simulink model "B3_2D_quadcopter_model"  (R2021b)
settings: Solver=VariableStepAuto  StartTime=0.0  StopTime=10  RelTol=1e-3
values from neighbouring files (symbols this model uses):
  omega_c_motors = 50    [A11_setup_script_pprz.m]    (also in A1_setup_script.m)
libraries: dspinverses x2, sim3dlib x1, uavsim3dlib x1, vrlib x1
settings Model: Creator=pieca  LastModifiedBy=pieca

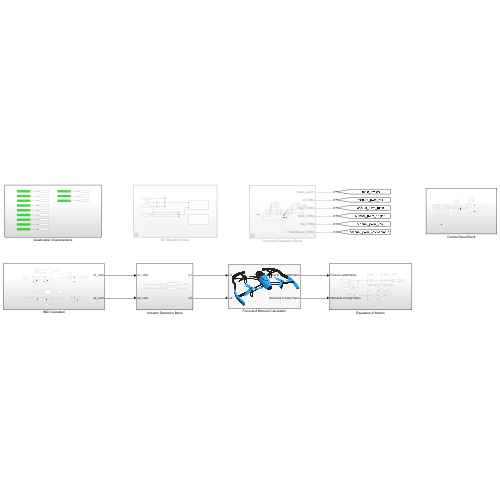
[thumbnail: Simulink's stored preview of the top-level diagram]
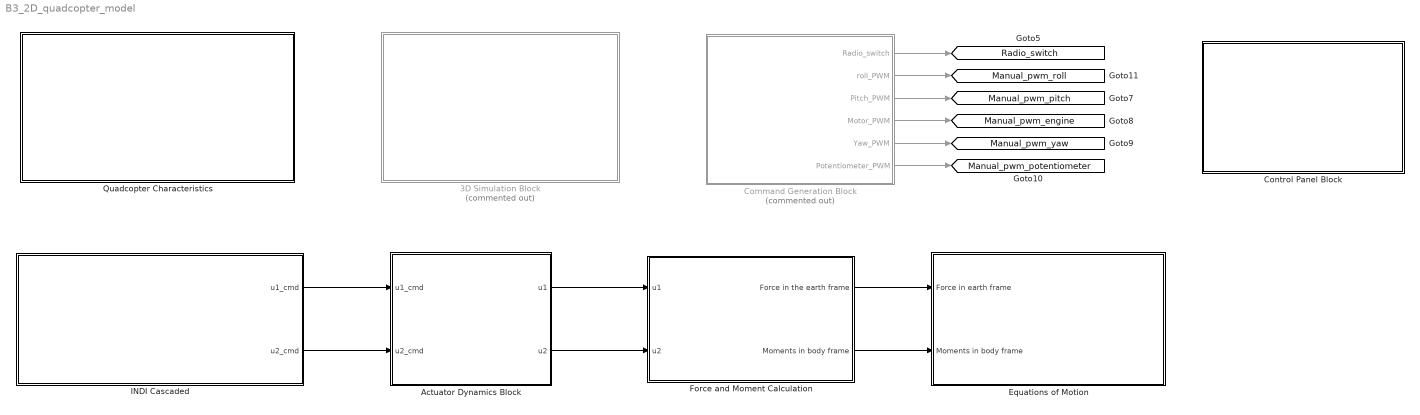
== system B3_2D_quadcopter_model ==
  3D Simulation Block : Subsystem  Commented=on
  Actuator Dynamics Block : Subsystem
  Command Generation Block : Subsystem  Commented=on
  Control Panel Block : Subsystem
  Equations of Motion : Subsystem
  Force and Moment Calculation : Subsystem
      mask Display: image('C:\Users\pieca\Desktop\AE5310-Thesis-Control\Quadcopter\media\bebop.jpg'); % Use "Edit Image" on toolstrip to change.
  INDI Cascaded : Subsystem
  Quadcopter Characteristics : Subsystem
  tag scope: Manual_pwm_engine=global, Manual_pwm_pitch=global, Manual_pwm_potentiometer=global, Manual_pwm_roll=global, Manual_pwm_yaw=global, Radio_switch=global
  wires:
  Command Generation Block/1(Radio_switch) -> [Radio_switch]
  Command Generation Block/2(roll_PWM) -> [Manual_pwm_roll]
  Command Generation Block/3(Pitch_PWM) -> [Manual_pwm_pitch]
  Command Generation Block/4(Motor_PWM) -> [Manual_pwm_engine]
  Command Generation Block/5(Yaw_PWM) -> [Manual_pwm_yaw]
  Command Generation Block/6(Potentiometer_PWM) -> [Manual_pwm_potentiometer]
  Force and Moment Calculation/1(Force in the earth frame) -> Equations of Motion/1(Force in earth frame)
  Force and Moment Calculation/2(Moments in body frame) -> Equations of Motion/2(Moments in body frame)
  Actuator Dynamics Block/1(u1) -> Force and Moment Calculation/1(u1)
  Actuator Dynamics Block/2(u2) -> Force and Moment Calculation/2(u2)
  INDI Cascaded/1(u1_cmd) -> Actuator Dynamics Block/1(u1_cmd)
  INDI Cascaded/2(u2_cmd) -> Actuator Dynamics Block/2(u2_cmd)

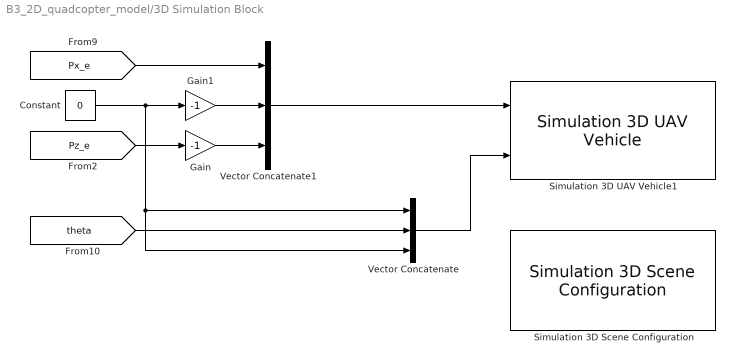
== system B3_2D_quadcopter_model/3D Simulation Block ==
  Constant : Constant  Value=0
  Gain : Gain  Gain=-1
  Gain1 : Gain  Gain=-1
  Simulation 3D Scene Configuration : sim3dlib/Simulation 3D Scene Configuration  Priority=0  ProjectFormat_internal=Default Scenes  ProjectFormat=Default Scenes  SceneDesc=US city block  ProjectName=C:\Program Files\MATLAB\R2021b\toolbox\shared\sim3d_projects\automotive_project\UE4\WindowsNoEditor\VehicleSimulation.exe  ScenePath=/Game/Maps/USCityBlock  vehTagList={'Scene Origin';'SimulinkVehicle1'}  vehTag=SimulinkVehicle1  OpVisEn=off  Ts=0.08  EnableWindow=on  EnableWeather=off  SunAltitude=40.0  SunAzimuth=90  clouds=10  wind=1  fog=0  rain=0  sensorTag=MainCamera1  sensorId=1  sensorName=MainCamera1  mountLoc=Origin  offsetFlag=off  tmountOffset=[0, 0, 0]  rmountOffset=[0, 0, 0]  HorizontalResolution=1280  VerticalResolution=720  HorizontalFOV=60  mountPoint=[0 0 0]  mountOrientation=[0 0 0]  aMode=4  ID=1
      settings: SourceProductBaseCode=AE,DR,UV,VE
  Simulation 3D UAV Vehicle1 : uavsim3dlib/Simulation 3D UAV Vehicle  Priority=-1  Mesh=Quadrotor  MeshPath=mesh\Fixed_Wing_UAV.stl  Color=Red  ActorName=SimulinkVehicle1  InitialTranslation=[0 0 0]  InitialRotation=[0 0 0]  SampleTime=-1  ActorType=SimulinkVehicle  ID=1  aMode=4  ActorTag=SimulinkVehicle1
      settings: SourceProductBaseCode=UV
  Vector Concatenate : Concatenate  NumInputs=3
  Vector Concatenate1 : Concatenate  NumInputs=3
  wires:
  Gain1/1 -> Vector Concatenate1/2
  [Px_e] -> Vector Concatenate1/1
  [Pz_e] -> Gain/1
  Gain/1 -> Vector Concatenate1/3
  Constant/1 -> Vector Concatenate/3, Vector Concatenate/1, Gain1/1
  [theta] -> Vector Concatenate/2
  Vector Concatenate1/1 -> Simulation 3D UAV Vehicle1/1
  Vector Concatenate/1 -> Simulation 3D UAV Vehicle1/2

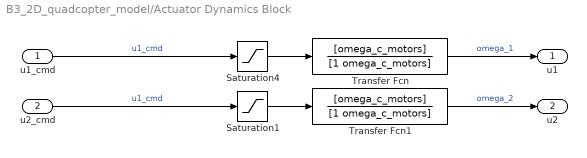
== system B3_2D_quadcopter_model/Actuator Dynamics Block ==
  u1_cmd : Inport
  u2_cmd : Inport  Port=2
  Saturation1 : Saturate  UpperLimit=10  LowerLimit=0
  Saturation4 : Saturate  UpperLimit=10  LowerLimit=0
  Transfer Fcn : TransferFcn  Numerator=[omega_c_motors]  Denominator=[1 omega_c_motors]
  Transfer Fcn1 : TransferFcn  Numerator=[omega_c_motors]  Denominator=[1 omega_c_motors]
  u1 : Outport
  u2 : Outport  Port=2
  wires:
  Saturation1/1 -> Transfer Fcn1/1
  Saturation4/1 -> Transfer Fcn/1
  u2_cmd/1 -> Saturation1/1  "u1_cmd"
  u1_cmd/1 -> Saturation4/1  "u1_cmd"
  Transfer Fcn1/1 -> u2/1  "omega_2"
  Transfer Fcn/1 -> u1/1  "omega_1"

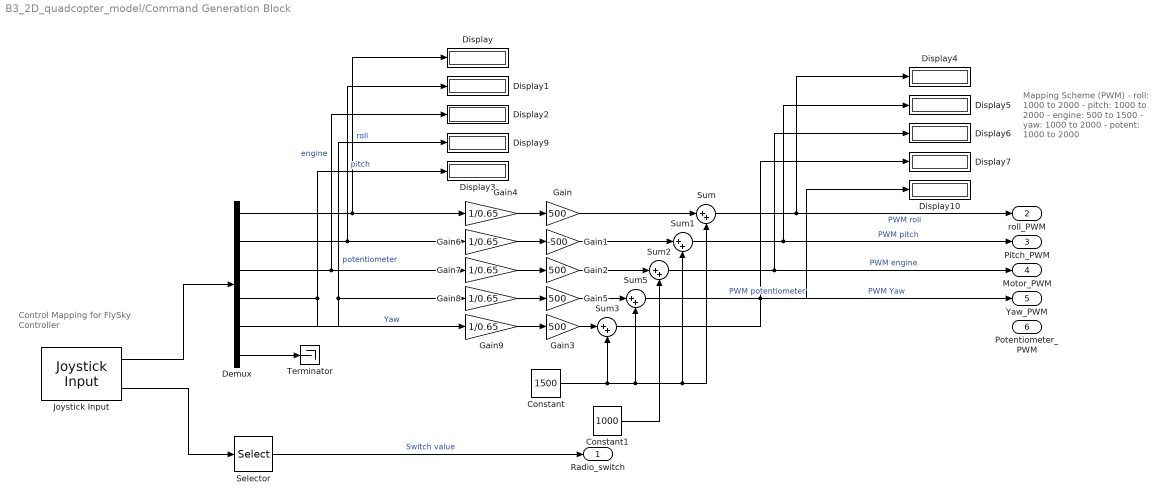
== system B3_2D_quadcopter_model/Command Generation Block ==
  note: Mapping Scheme (PWM)
      |
      | - roll: 1000 to 2000
      | - pitch: 1000 to 2000
      | - engine: 500 to 1500
      | - yaw: 1000 to 2000
      | - potent: 1000 to 2000
  note: Control Mapping for FlySky Controller
  Constant : Constant  Value=1500
  Constant1 : Constant  Value=1000
  Demux : Demux  Outputs=6
  Display{,1..7,9..10} (10 alike) : Display
  Gain{,2..3,5} (4 alike) : Gain  Gain=500
  Gain1 : Gain  Gain=-500
  Gain{4,6..9} (5 alike) : Gain  Gain=1/0.65
  Joystick Input : vrlib/Joystick Input  joyid=1  adjustports=on  forcefeed=off
  Selector : Selector  InputPortWidth=16  IndexOptions=Index vector (dialog)  Indices=1  OutputSizes=1
  Sum{,1..3,5} (5 alike) : Sum  Inputs=|++
  Terminator : Terminator
  Radio_switch : Outport
  roll_PWM : Outport  Port=2
  Pitch_PWM : Outport  Port=3
  Motor_PWM : Outport  Port=4
  Yaw_PWM : Outport  Port=5
  Potentiometer_PWM : Outport  Port=6
  wires:
  Gain2/1 -> Sum2/1
  Joystick Input/2 -> Selector/1
  Gain1/1 -> Sum1/1
  Sum/1 -> roll_PWM/1, Display4/1  "PWM roll"
  Constant1/1 -> Sum2/2
  Selector/1 -> Radio_switch/1  "Switch value"
  Gain5/1 -> Sum5/1
  Joystick Input/1 -> Demux/1
  Sum3/1 -> Yaw_PWM/1, Display7/1  "PWM Yaw"
  Sum5/1 -> Display10/1  "PWM potentiometer"
  Demux/1 -> Display/1, Gain4/1  "roll"
  Demux/2 -> Gain6/1, Display1/1  "pitch"
  Demux/5 -> Gain8/1, Display9/1  "potentiometer"
  Constant/1 -> Sum5/2, Sum/2, Sum1/2, Sum3/2
  Sum2/1 -> Motor_PWM/1, Display6/1  "PWM engine"
  Sum1/1 -> Pitch_PWM/1, Display5/1  "PWM pitch"
  Gain/1 -> Sum/1
  Demux/4 -> Gain9/1, Display3/1  "Yaw"
  Gain3/1 -> Sum3/1
  Demux/3 -> Gain7/1, Display2/1  "engine"
  Demux/6 -> Terminator/1
  Gain6/1 -> Gain1/1
  Gain9/1 -> Gain3/1
  Gain7/1 -> Gain2/1
  Gain4/1 -> Gain/1
  Gain8/1 -> Gain5/1

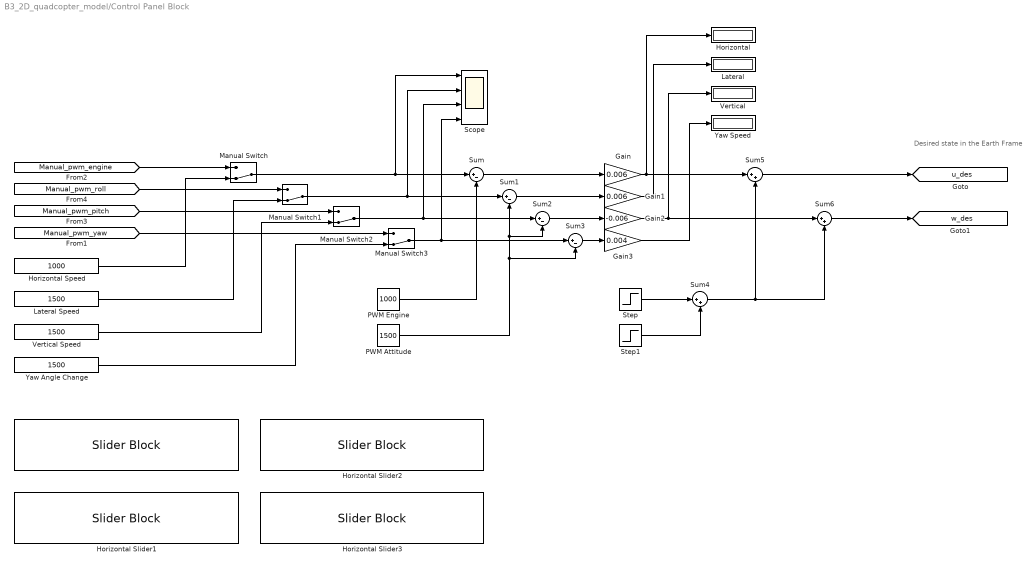
== system B3_2D_quadcopter_model/Control Panel Block ==
  note: Desired state in the Earth Frame
  " " : SliderBlock  ScaleMin=500  ScaleMax=1500
  Gain : Gain  Gain=0.006
  Gain1 : Gain  Gain=0.006
  Gain2 : Gain  Gain=-0.006
  Gain3 : Gain  Gain=0.004
  Horizontal : Display
  Horizontal Slider1 : SliderBlock  ScaleMin=1000  ScaleMax=2000
  Horizontal Slider2 : SliderBlock  ScaleMin=1000  ScaleMax=2000
  Horizontal Slider3 : SliderBlock  ScaleMin=1000  ScaleMax=2000
  Horizontal Speed : Constant  Value=1000
  Lateral : Display
  Lateral Speed : Constant  Value=1500
  Manual Switch{,1..3} (4 alike) : ManualSwitch  CurrentSetting=0
  PWM Attitude : Constant  Value=1500
  PWM Engine : Constant  Value=1000
  Scope : Scope  NumInputPorts=4
  Step : Step  Time=3  After=5  SampleTime=0
  Step1 : Step  Time=7  After=-5  SampleTime=0
  Sum{,1..3} (4 alike) : Sum  Inputs=|+-
  Sum4 : Sum  Inputs=|++
  Sum5 : Sum  Inputs=|++
  Sum6 : Sum  Inputs=|++
  Vertical : Display
  Vertical Speed : Constant  Value=1500
  Yaw Angle Change : Constant  Value=1500
  Yaw Speed : Display
  tag scope: u_des=global, w_des=global
  wires:
  [Manual_pwm_roll] -> Manual Switch1/1
  Manual Switch3/1 -> Scope/4, Sum3/1
  [Manual_pwm_yaw] -> Manual Switch3/1
  Sum/1 -> Gain/1
  Gain/1 -> Sum5/1, Horizontal/1
  PWM Attitude/1 -> Sum3/2, Sum2/2, Sum1/2
  Horizontal Speed/1 -> Manual Switch/2
  Sum1/1 -> Gain1/1
  Yaw Angle Change/1 -> Manual Switch3/2
  Lateral Speed/1 -> Manual Switch1/2
  Vertical Speed/1 -> Manual Switch2/2
  Manual Switch/1 -> Scope/1, Sum/1
  Manual Switch1/1 -> Scope/2, Sum1/1
  Manual Switch2/1 -> Scope/3, Sum2/1
  Sum2/1 -> Gain2/1
  Sum3/1 -> Gain3/1
  Gain2/1 -> Sum6/1, Vertical/1
  [Manual_pwm_engine] -> Manual Switch/1
  [Manual_pwm_pitch] -> Manual Switch2/1
  PWM Engine/1 -> Sum/2
  Gain1/1 -> Lateral/1
  Gain3/1 -> Yaw Speed/1
  Step1/1 -> Sum4/2
  Step/1 -> Sum4/1
  Sum6/1 -> [w_des]
  Sum5/1 -> [u_des]
  Sum4/1 -> Sum6/2, Sum5/2

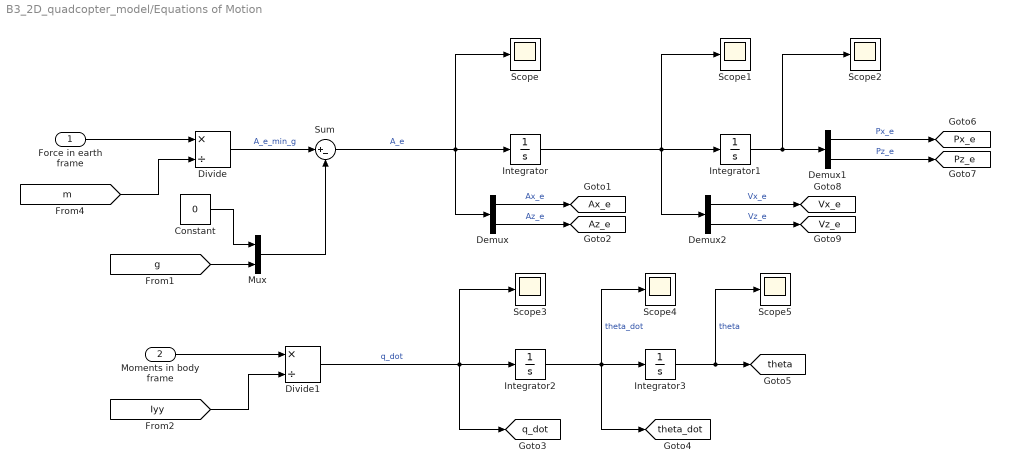
== system B3_2D_quadcopter_model/Equations of Motion ==
  Force in earth frame : Inport
  Moments in body frame : Inport  Port=2
  Constant : Constant  Value=0
  Demux : Demux  Outputs=2
  Demux1 : Demux  Outputs=2
  Demux2 : Demux  Outputs=2
  Divide : Product  Inputs=*/
  Divide1 : Product  Inputs=*/
  Integrator{,1..3} (4 alike) : Integrator
  Mux : Mux  Inputs=2
  Scope{,1..5} (6 alike) : Scope
  Sum : Sum  Inputs=|+-
  tag scope: Ax_e=global, Az_e=global, Px_e=global, Pz_e=global, Vx_e=global, Vz_e=global, q_dot=global, theta=global, theta_dot=global
  wires:
  Force in earth frame/1 -> Divide/1
  [m] -> Divide/2
  Sum/1 -> Scope/1, Demux/1, Integrator/1  "A_e"
  Integrator/1 -> Scope1/1, Demux2/1, Integrator1/1
  Integrator1/1 -> Scope2/1, Demux1/1
  Moments in body frame/1 -> Divide1/1
  [Iyy] -> Divide1/2
  Divide1/1 -> Scope3/1, [q_dot], Integrator2/1  "q_dot"
  Integrator2/1 -> Scope4/1, [theta_dot], Integrator3/1  "theta_dot"
  Integrator3/1 -> Scope5/1, [theta]  "theta"
  Demux/1 -> [Ax_e]  "Ax_e"
  Demux/2 -> [Az_e]  "Az_e"
  Demux1/2 -> [Pz_e]  "Pz_e"
  Demux1/1 -> [Px_e]  "Px_e"
  Demux2/2 -> [Vz_e]  "Vz_e"
  Demux2/1 -> [Vx_e]  "Vx_e"
  Divide/1 -> Sum/1  "A_e_min_g"
  [g] -> Mux/2
  Mux/1 -> Sum/2
  Constant/1 -> Mux/1

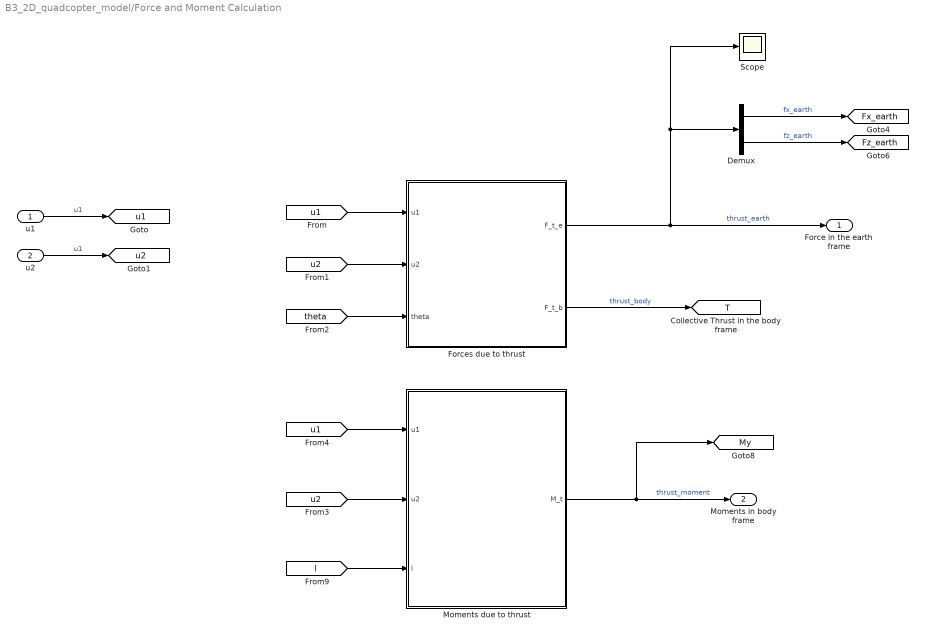
== system B3_2D_quadcopter_model/Force and Moment Calculation ==
  u1 : Inport
  u2 : Inport  Port=2
  Demux : Demux  Outputs=2
  Forces due to thrust : MATLAB Function  TreatAsAtomicUnit=on
  Moments due to thrust : MATLAB Function  TreatAsAtomicUnit=on
  Scope : Scope
  Force in the earth frame : Outport
  Moments in body frame : Outport  Port=2
  tag scope: Fx_earth=global, Fz_earth=global, My=global, T=global, u1=global, u2=global
  wires:
  u1/1 -> [u1]  "u1"
  u2/1 -> [u2]  "u1"
  Forces due to thrust/1(F_t_e) -> Scope/1, Demux/1, Force in the earth frame/1  "thrust_earth"
  Demux/1 -> [Fx_earth]  "fx_earth"
  Demux/2 -> [Fz_earth]  "fz_earth"
  Forces due to thrust/2(F_t_b) -> [T]  "thrust_body"
  [l] -> Moments due to thrust/3(l)
  [theta] -> Forces due to thrust/3(theta)
  [u2] -> Forces due to thrust/2(u2)
  [u1] -> Forces due to thrust/1(u1)
  [u1] -> Moments due to thrust/1(u1)
  [u2] -> Moments due to thrust/2(u2)
  Moments due to thrust/1(M_t) -> [My], Moments in body frame/1  "thrust_moment"

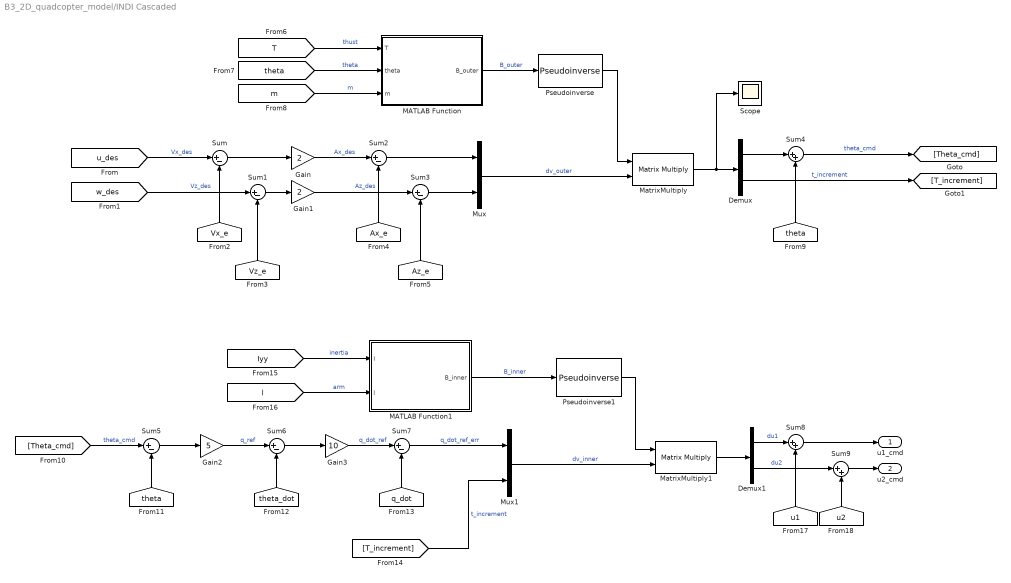
== system B3_2D_quadcopter_model/INDI Cascaded ==
  Demux : Demux  Outputs=2
  Demux1 : Demux  Outputs=2
  Gain : Gain  Gain=2
  Gain1 : Gain  Gain=2
  Gain2 : Gain  Gain=5
  Gain3 : Gain  Gain=10
  MATLAB Function : MATLAB Function  TreatAsAtomicUnit=on
  MATLAB Function1 : MATLAB Function  TreatAsAtomicUnit=on
  MatrixMultiply : Product  Multiplication=Matrix(*)
  MatrixMultiply1 : Product  Multiplication=Matrix(*)
  Mux : Mux  Inputs=2
  Mux1 : Mux  Inputs=2
  Pseudoinverse : dspinverses/Pseudoinverse  wanterr=off  SimulateUsing=Interpreted execution
      settings: SourceProductBaseCode=DS
  Pseudoinverse1 : dspinverses/Pseudoinverse  wanterr=off  SimulateUsing=Interpreted execution
      settings: SourceProductBaseCode=DS
  Scope : Scope
  Sum{,1..3,5..7} (7 alike) : Sum  Inputs=|+-
  Sum4 : Sum  Inputs=|++
  Sum8 : Sum  Inputs=|++
  Sum9 : Sum  Inputs=|++
  u1_cmd : Outport
  u2_cmd : Outport  Port=2
  wires:
  [u_des] -> Sum/1  "Vx_des"
  [w_des] -> Sum1/1  "Vz_des"
  Sum/1 -> Gain/1
  Sum1/1 -> Gain1/1
  [Vx_e] -> Sum/2
  [Vz_e] -> Sum1/2
  Sum3/1 -> Mux/2
  Gain1/1 -> Sum3/1  "Az_des"
  Sum2/1 -> Mux/1
  Gain/1 -> Sum2/1  "Ax_des"
  [Az_e] -> Sum3/2
  [Ax_e] -> Sum2/2
  Mux/1 -> MatrixMultiply/2  "dv_outer"
  [T] -> MATLAB Function/1(T)  "thust"
  [m] -> MATLAB Function/3(m)  "m"
  [theta] -> MATLAB Function/2(theta)  "theta"
  MATLAB Function/1(B_outer) -> Pseudoinverse/1  "B_outer"
  Pseudoinverse/1 -> MatrixMultiply/1
  MatrixMultiply/1 -> Scope/1, Demux/1
  Demux/1 -> Sum4/1
  Sum4/1 -> [Theta_cmd]  "theta_cmd"
  Demux/2 -> [T_increment]  "t_increment"
  [theta] -> Sum4/2
  [Theta_cmd] -> Sum5/1  "theta_cmd"
  Sum5/1 -> Gain2/1
  Sum6/1 -> Gain3/1
  Gain2/1 -> Sum6/1  "q_ref"
  [theta] -> Sum5/2
  [theta_dot] -> Sum6/2
  Gain3/1 -> Sum7/1  "q_dot_ref"
  [q_dot] -> Sum7/2
  Sum7/1 -> Mux1/1  "q_dot_ref_err"
  [T_increment] -> Mux1/2  "t_increment"
  Pseudoinverse1/1 -> MatrixMultiply1/1
  Mux1/1 -> MatrixMultiply1/2  "dv_inner"
  [Iyy] -> MATLAB Function1/1(I)  "inertia"
  [l] -> MATLAB Function1/2(l)  "arm"
  MATLAB Function1/1(B_inner) -> Pseudoinverse1/1  "B_inner"
  MatrixMultiply1/1 -> Demux1/1
  Sum8/1 -> u1_cmd/1
  Demux1/1 -> Sum8/1  "du1"
  Sum9/1 -> u2_cmd/1
  Demux1/2 -> Sum9/1  "du2"
  [u1] -> Sum8/2
  [u2] -> Sum9/2

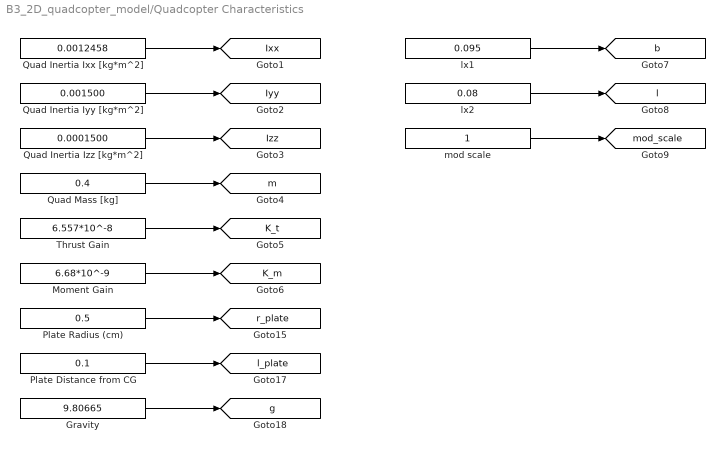
== system B3_2D_quadcopter_model/Quadcopter Characteristics ==
  Gravity : Constant  Value=9.80665
  Moment Gain : Constant  Value=6.68*10^-9
  Plate Distance from CG : Constant  Value=0.1
  Plate Radius (cm) : Constant  Value=0.5
  Quad Inertia Ixx [kg*m^2] : Constant  Value=0.0012458
  Quad Inertia Iyy [kg*m^2] : Constant  Value=0.001500
  Quad Inertia Izz [kg*m^2] : Constant  Value=0.0001500
  Quad Mass [kg] : Constant  Value=0.4
  Thrust Gain : Constant  Value=6.557*10^-8
  lx1 : Constant  Value=0.095
  lx2 : Constant  Value=0.08
  mod scale : Constant
  tag scope: Ixx=global, Iyy=global, Izz=global, K_m=global, K_t=global, b=global, g=global, l=global, l_plate=global, m=global, mod_scale=global, r_plate=global
  wires:
  Quad Inertia Ixx [kg*m^2]/1 -> [Ixx]
  Quad Inertia Iyy [kg*m^2]/1 -> [Iyy]
  Quad Inertia Izz [kg*m^2]/1 -> [Izz]
  Quad Mass [kg]/1 -> [m]
  Thrust Gain/1 -> [K_t]
  Moment Gain/1 -> [K_m]
  lx1/1 -> [b]
  lx2/1 -> [l]
  Plate Radius (cm)/1 -> [r_plate]
  Plate Distance from CG/1 -> [l_plate]
  Gravity/1 -> [g]
  mod scale/1 -> [mod_scale]

== matlab function B3_2D_quadcopter_model/INDI Cascaded/MATLAB Function ==
  data: T input; B_outer output; theta input; m input
function B_outer = B_outer_loop(T,theta,m)

B_outer = zeros(2,2);

B_outer(1,1) = T*cos(theta)*(1/m);  
B_outer(1,2) = sin(theta)*(1/m);
B_outer(2,1) = -T*sin(theta)*(1/m);
B_outer(2,2) = cos(theta)*(1/m);

== matlab function B3_2D_quadcopter_model/Force and Moment Calculation/Forces due to thrust ==
  data: u1 input; u2 input; F_t_e output; theta input; F_t_b output
function [F_t_e, F_t_b] = F_t(u1, u2, theta)

F_t_b = u1+u2;
F_t_e = zeros(2,1);

F_t_e(1,1) = F_t_b*sin(theta);
F_t_e(2,1) = F_t_b*cos(theta);

== matlab function B3_2D_quadcopter_model/Force and Moment Calculation/Moments due to thrust ==
  data: u1 input; u2 input; M_t output; l input
function M_t = M_t(u1,u2,l)

M_t = l*(u1-u2);

== matlab function B3_2D_quadcopter_model/INDI Cascaded/MATLAB Function1 ==
  data: I input; B_inner output; l input
function B_inner = B_inner_loop(I,l)

B_inner = zeros(2,2);

B_inner(1,1) = l/I;  
B_inner(1,2) = -l/I;
B_inner(2,1) = 1;
B_inner(2,2) = 1;
